simulink model "AdaptiveInverseDynamicsControl"  (R2021a)
settings: Solver=FixedStepAuto  StartTime=0.0  StopTime=5  FixedStep=0.001  RelTol=1e-3
InitFcn:
  | gamma = 0.00001*[1 0 0 0 0 0 0 0 0; 0 1 0 0 0 0 0 0 0; 0 0 1 0 0 0 0 0 0; 0 0 0 1 0 0 0 0 0; 0 0 0 0 1 0 0 0 0; 0 0 0 0 0 1 0 0 0; 0 0 0 0 0 0 1 0 0; 0 0 0 0 0 0 0 1 0; 0 0 0 0 0 0 0 0 1];
  | P = [-49 0 0 53 0 0; 0 -49 0 0 53 0; 0 0 -49 0 0 53; 53 0 0 -59 0 0; 0 53 0 0 -59 0; 0 0 53 0 0 -59];
  | kd1 = 60;
  | kd2 = 60;
  | kd3 = 60;
  | kp1 = 60;
  | kp2 = 60;
  | kp3 = 60;
  | Mhat = [3.5 0 0; 0 3.5 0.75; 0 0.75 1.25];
  | theta = [1.25; 0.25; 0.5; 1; 1; 1; 1; 1; 1];
libraries: aerolibutil x1
settings Model: Creator=negin  LastModifiedBy=negin

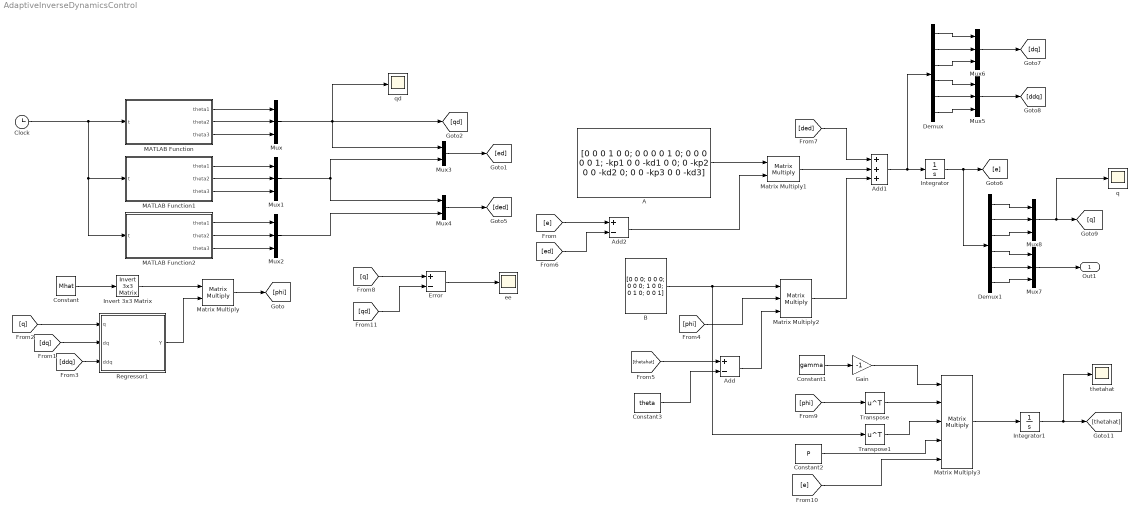
== system AdaptiveInverseDynamicsControl ==
  A : Constant  Value=[0 0 0 1 0 0; 0 0 0 0 1 0; 0 0 0 0 0 1; -kp1 0 0 -kd1 0 0; 0 -kp2 0 0 -kd2 0; 0 0 -kp3 0 0 -kd3]
  Add : Sum  Inputs=+-
  Add1 : Sum  Inputs=+++
  Add2 : Sum  Inputs=+-
  B : Constant  Value=[0 0 0; 0 0 0; 0 0 0; 1 0 0; 0 1 0; 0 0 1]
  Clock : Clock
      settings: Decimation=5
  Constant : Constant  Value=Mhat  VectorParams1D=off
  Constant1 : Constant  Value=gamma  VectorParams1D=off
  Constant2 : Constant  Value=P  VectorParams1D=off
  Constant3 : Constant  Value=theta  VectorParams1D=off
  Demux : Demux  Outputs=6
  Demux1 : Demux  Outputs=6
  Error : Sum  Inputs=+-
  Gain : Gain  Gain=-1
  Integrator : Integrator  InitialCondition=[0; 0; 0; 0; 0; 0]
  Integrator1 : Integrator  InitialCondition=[1.25; 0.25; 0.5; 1; 1; 1; 1; 1; 1].*1.05
  Invert 3x3 Matrix : aerolibutil/Invert  3x3 Matrix
  MATLAB Function : MATLAB Function  TreatAsAtomicUnit=on
  MATLAB Function1 : MATLAB Function  TreatAsAtomicUnit=on
  MATLAB Function2 : MATLAB Function  TreatAsAtomicUnit=on
  Matrix Multiply : Product  Multiplication=Matrix(*)
  Matrix Multiply1 : Product  Multiplication=Matrix(*)
  Matrix Multiply2 : Product  Inputs=3  Multiplication=Matrix(*)
  Matrix Multiply3 : Product  Inputs=5  Multiplication=Matrix(*)
  Mux{,1..2,5..8} (7 alike) : Mux  Inputs=3
  Mux3 : Mux  Inputs=2
  Mux4 : Mux  Inputs=2
  Regressor1 : MATLAB Function  TreatAsAtomicUnit=on
  Transpose : Math  Operator=transpose  SaturateOnIntegerOverflow=on
  Transpose1 : Math  Operator=transpose  SaturateOnIntegerOverflow=on
  ee : Scope
  q : Scope
  qd : Scope
  thetahat : Scope
  Out1 : Outport
  wires:
  MATLAB Function/1(theta1) -> Mux/1
  Clock/1 -> MATLAB Function/1(t), MATLAB Function1/1(t), MATLAB Function2/1(t)
  MATLAB Function/2(theta2) -> Mux/2
  MATLAB Function/3(theta3) -> Mux/3
  Mux/1 -> qd/1, [qd], Mux3/1
  MATLAB Function1/1(theta1) -> Mux1/1
  MATLAB Function1/2(theta2) -> Mux1/2
  MATLAB Function1/3(theta3) -> Mux1/3
  MATLAB Function2/1(theta1) -> Mux2/1
  MATLAB Function2/2(theta2) -> Mux2/2
  MATLAB Function2/3(theta3) -> Mux2/3
  Mux1/1 -> Mux4/1, Mux3/2
  Mux2/1 -> Mux4/2
  [dq] -> Regressor1/2(dq)
  [q] -> Regressor1/1(q)
  [ddq] -> Regressor1/3(ddq)
  Constant/1 -> Invert 3x3 Matrix/1
  Invert 3x3 Matrix/1 -> Matrix Multiply/1
  Regressor1/1(Y) -> Matrix Multiply/2
  Matrix Multiply/1 -> [phi]
  A/1 -> Matrix Multiply1/1
  [thetahat] -> Add/1
  Constant3/1 -> Add/2
  B/1 -> Transpose1/1, Matrix Multiply2/1
  [phi] -> Matrix Multiply2/2
  Add/1 -> Matrix Multiply2/3
  Mux3/1 -> [ed]
  [e] -> Add2/1
  [ed] -> Add2/2
  Add2/1 -> Matrix Multiply1/2
  Matrix Multiply2/1 -> Add1/3
  Matrix Multiply1/1 -> Add1/2
  Mux4/1 -> [ded]
  [ded] -> Add1/1
  Add1/1 -> Demux/1, Integrator/1
  Integrator/1 -> Demux1/1, [e]
  Demux/4 -> Mux5/1
  Demux/5 -> Mux5/2
  Demux/6 -> Mux5/3
  Demux/1 -> Mux6/1
  Demux/2 -> Mux6/2
  Demux/3 -> Mux6/3
  Mux6/1 -> [dq]
  Mux5/1 -> [ddq]
  Demux1/4 -> Mux7/1
  Mux8/1 -> q/1, [q]
  Demux1/5 -> Mux7/2
  Demux1/3 -> Mux8/3
  Demux1/2 -> Mux8/2
  Demux1/6 -> Mux7/3
  Mux7/1 -> Out1/1
  Demux1/1 -> Mux8/1
  [phi] -> Transpose/1
  Constant1/1 -> Gain/1
  Gain/1 -> Matrix Multiply3/1
  Transpose/1 -> Matrix Multiply3/2
  Transpose1/1 -> Matrix Multiply3/3
  Constant2/1 -> Matrix Multiply3/4
  [e] -> Matrix Multiply3/5
  Matrix Multiply3/1 -> Integrator1/1
  Integrator1/1 -> thetahat/1, [thetahat]
  [q] -> Error/1
  [qd] -> Error/2
  Error/1 -> ee/1

== matlab function AdaptiveInverseDynamicsControl/MATLAB Function ==
  data: theta1 output; t input; theta2 output; theta3 output
function [theta1, theta2, theta3] = desiredTraj(t)
theta1 = 0.1309*t^2 + 0.0147*t^3 - 0.0085*t^4 + 0.0007*t^5;
theta2 = 0.1309*t^2 - 0.0188*t^3 - 0.001*t^4 + 0.0002*t^5;
theta3 = 0.1309*t^2 + 0.0314*t^3 - 0.0123*t^4 + 0.001*t^5;

== matlab function AdaptiveInverseDynamicsControl/Regressor1 ==
  data: q input; Y output; dq input; ddq input
function Y = RegressorMatrix(q, dq, ddq)

% m1 = 1;
% m2 = 1;
% m3 = 1;
% 
% l1 = 1;
% l2 = 1;
% l3 = 1;
% 
% r1 = l1/2;
% r2 = l2/2;
% r3 = l3/2;
% 
% R1 = 0.05;
% R2 = 0.05;
% R3 = 0.05;
% 
 g = 9.81;
% 
% a1 = m2*r2^2 + m3*l2^2;
% a2 = m3*r3^2;
% a3 = m3*r3*l2;
% b1 = (m2*r2 + m3*l2)*g;
% b2 = m3*r3*g;
% I1 = 0.5*m1*R1^2;
% I2 = 0.5*m2*R2^2;
% I3 = 0.5*m3*R3^2;


M = [cos(q(2))^2*ddq(1), cos(q(2) + q(3))^2*ddq(1), 2*cos(q(2))*cos(q(2) + q(3))*ddq(1), ddq(1), 0, 0, 0, 0, 0;...
    ddq(2), ddq(2) + ddq(3), 2*cos(q(3))*ddq(2) + ddq(3)*cos(q(3)), 0, ddq(2), 0, 0, 0, 0;...
    0, ddq(2) + ddq(3), ddq(2)*cos(q(3)), 0, 0, ddq(3), 0, 0, 0];

C = [-0.5*dq(2)*sin(2*q(2))*dq(1) - 0.5*dq(2)*dq(1)*sin(2*q(2)), - 0.5*(dq(2) + dq(3))*sin(2*q(2) + 2*q(3))*dq(1)...
    - 0.5*dq(2)*dq(1)*sin(2*q(2) + 2*q(3)) - 0.5*dq(3)*dq(1)*sin(2*q(2) + 2*q(3)), - dq(2)*sin(2*q(2) + q(3))*dq(1)...
    - dq(1)*dq(3)*cos(q(2))*sin(q(2) + q(3)) - dq(2)*dq(1)*sin(2*q(2) + q(3)) - dq(3)*dq(1)*cos(q(2))*sin(q(2) + q(3))...
    , 0, 0, 0, 0, 0, 0;...
    0.5*dq(1)*dq(1)*sin(2*q(2)), 0.5*dq(1)*dq(1)*sin(2*q(2) + 2*q(3)), dq(1)*dq(1)*sin(2*q(2) + q(3)) - dq(2)*dq(3)...
    *sin(q(3)) - dq(3)*(dq(2) + dq(3))*sin(q(3)), 0, 0, 0, 0, 0, 0;...
    0, 0.5*dq(1)*dq(1)*sin(2*q(2) + 2*q(3)), dq(1)*dq(1)*cos(q(2))*sin(q(2) + q(3)) + dq(2)*dq(2)*sin(q(3)),...
    0, 0, 0, 0, 0, 0];

G = [0, 0, 0, 0, 0, 0, 0, 0, 0; ...
    0, 0, 0, 0, 0, 0, sin(q(2))*g/2, - sin(q(2) + q(3))*g/2, - sin(q(2))*g; ...
    0, 0, 0, 0, 0, 0, 0, -sin(q(2) + q(3))*g/2, 0];

Y = M + C + G;
%theta = [a1; a2; a3; I1; I2; I3; m2*l2; m3*l3; m3*l2];

end

== matlab function AdaptiveInverseDynamicsControl/MATLAB Function1 ==
  data: theta1 output; t input; theta2 output; theta3 output
function [theta1, theta2, theta3] = ddesiredTraj(t)
theta1 = 0.1309*2*t + 0.0147*3*t^2 - 0.0085*4*t^3 + 0.0007*5*t^4;
theta2 = 0.1309*2*t - 0.0188*3*t^2 - 0.001*4*t^3 + 0.0002*5*t^4;
theta3 = 0.1309*2*t + 0.0314*3*t^2 - 0.0123*4*t^3 + 0.001*5*t^4;

== matlab function AdaptiveInverseDynamicsControl/MATLAB Function2 ==
  data: theta1 output; t input; theta2 output; theta3 output
function [theta1, theta2, theta3] = dddesiredTraj(t)
theta1 = 0.1309*2 + 0.0147*3*2*t - 0.0085*4*3*t^2 + 0.0007*5*4*t^3;
theta2 = 0.1309*2 - 0.0188*3*2*t - 0.001*4*3*t^2 + 0.0002*5*4*t^3;
theta3 = 0.1309*2 + 0.0314*3*2*t - 0.0123*4*3*t^2 + 0.001*5*4*t^3;
